simulink model "Scenario_3_PF"  (R2020b)
settings: Solver=ode1  StartTime=0.0  StopTime=10.0  RelTol=1e-3
InitFcn:
  | Scenario_3_parameters;
values from neighbouring files (symbols this model uses):
  c0 = c0_zeb    (= 6.57988e-09)    [Scenario_17_parameters_v2.m]    (also in Scenario_1_parameters_v2.m; Scenario_2_parameters_v2.m; Scenario_3_parameters_v2.m)
  c0_hawk = 6.37282e-09    [Scenario_17_parameters_v2.m]    (also in Scenario_1_parameters_v2.m; Scenario_2_parameters_v2.m; Scenario_3_parameters_v2.m)
  c1 = c1_zeb    (= 9.15905e-09)    [Scenario_17_parameters_v2.m]    (also in Scenario_1_parameters_v2.m; Scenario_2_parameters_v2.m; Scenario_3_parameters_v2.m)
  c1_hawk = 8.76156e-09    [Scenario_17_parameters_v2.m]    (also in Scenario_1_parameters_v2.m; Scenario_2_parameters_v2.m; Scenario_3_parameters_v2.m)
  fg = 50    [Scenario_17_parameters_v2.m]    (also in Scenario_1_parameters_v2.m; Scenario_2_parameters_v2.m; Scenario_3_parameters_v2.m)
  G10gen = 0.90    (= 0.9)    [Scenario_3_parameters_v2.m]
  G12gen = 0.85    [Scenario_3_parameters_v2.m]
  G1gen = 0.4692    [Scenario_17_parameters_v2.m]    (also in Scenario_1_parameters_v2.m = 0.1; Scenario_2_parameters_v2.m = 0.298581; Scenario_3_parameters_v2.m = 0.65)
  G2gen = 0.80    (= 0.8)    [Scenario_1_parameters_v2.m]    (also in Scenario_2_parameters_v2.m = 0.7; Scenario_3_parameters_v2.m = 0.4)
  G3gen = 0.85    [Scenario_1_parameters_v2.m]    (also in Scenario_2_parameters_v2.m = 0.9; Scenario_3_parameters_v2.m = 0.6)
  G4gen = 0.65    [Scenario_3_parameters_v2.m]
  G5gen = 0.75    [Scenario_17_parameters_v2.m]    (also in Scenario_1_parameters_v2.m = 0.8; Scenario_2_parameters_v2.m = 0.8; Scenario_3_parameters_v2.m = 0.705)
  G6gen = 0.90    (= 0.9)    [Scenario_17_parameters_v2.m]    (also in Scenario_1_parameters_v2.m; Scenario_2_parameters_v2.m = 0.81797; Scenario_3_parameters_v2.m = 0.45)
  G7gen = 0.20    (= 0.2)    [Scenario_17_parameters_v2.m]    (also in Scenario_1_parameters_v2.m = 0.5227; Scenario_2_parameters_v2.m = 0.5098; Scenario_3_parameters_v2.m = 0.4)
  G8gen = 0.58    [Scenario_17_parameters_v2.m]    (also in Scenario_3_parameters_v2.m = 0.65)
  G9gen = 0.8833    [Scenario_17_parameters_v2.m]    (also in Scenario_3_parameters_v2.m = 0.9)
  Ihvpk = Ihv*sqrt(2)    [Scenario_17_parameters_v2.m]    (also in Scenario_1_parameters_v2.m; Scenario_2_parameters_v2.m; Scenario_3_parameters_v2.m)
  l0 = l0_zeb    (= 0.00368)    [Scenario_17_parameters_v2.m]    (also in Scenario_1_parameters_v2.m; Scenario_2_parameters_v2.m; Scenario_3_parameters_v2.m)
  l0_hawk = 0.00373    [Scenario_17_parameters_v2.m]    (also in Scenario_1_parameters_v2.m; Scenario_2_parameters_v2.m; Scenario_3_parameters_v2.m)
  l1 = l1_zeb    (= 0.00128)    [Scenario_17_parameters_v2.m]    (also in Scenario_1_parameters_v2.m; Scenario_2_parameters_v2.m; Scenario_3_parameters_v2.m)
  L10dem = 0.04    [Scenario_3_parameters_v2.m]
  L12dem = 0.01    [Scenario_17_parameters_v2.m]    (also in Scenario_3_parameters_v2.m = 0.02)
  L13dem = 0.01    [Scenario_3_parameters_v2.m]
  l1_hawk = 0.00133    [Scenario_17_parameters_v2.m]    (also in Scenario_1_parameters_v2.m; Scenario_2_parameters_v2.m; Scenario_3_parameters_v2.m)
  L1dem = 0.25    [Scenario_17_parameters_v2.m]    (also in Scenario_3_parameters_v2.m = 0.1)
  L3dem = 0.30    (= 0.3)    [Scenario_17_parameters_v2.m]    (also in Scenario_1_parameters_v2.m = 0.1; Scenario_2_parameters_v2.m = 0.1; Scenario_3_parameters_v2.m = 0.2)
  L6dem = 0.15    [Scenario_1_parameters_v2.m]    (also in Scenario_2_parameters_v2.m; Scenario_3_parameters_v2.m = 0.1)
  L7dem = 0.10    (= 0.1)    [Scenario_1_parameters_v2.m]    (also in Scenario_2_parameters_v2.m; Scenario_3_parameters_v2.m = 0.2)
  L9dem = 0.15    [Scenario_17_parameters_v2.m]    (also in Scenario_3_parameters_v2.m = 0.1)
  Pr = Sr*PF    (= 1600500000)    [Scenario_17_parameters_v2.m]    (also in Scenario_1_parameters_v2.m = 1472500000; Scenario_2_parameters_v2.m = 1805000000; Scenario_3_parameters_v2.m = 12740000000)
  Qr = sqrt(Sr^2 - Pr^2)    [Scenario_17_parameters_v2.m]    (also in Scenario_1_parameters_v2.m; Scenario_2_parameters_v2.m; Scenario_3_parameters_v2.m)
  r0 = r0_zeb    (= 0.39362)    [Scenario_17_parameters_v2.m]    (also in Scenario_1_parameters_v2.m; Scenario_2_parameters_v2.m; Scenario_3_parameters_v2.m)
  r0_hawk = 0.44587    [Scenario_17_parameters_v2.m]    (also in Scenario_1_parameters_v2.m; Scenario_2_parameters_v2.m; Scenario_3_parameters_v2.m)
  r1 = r1_zeb    (= 0.06862)    [Scenario_17_parameters_v2.m]    (also in Scenario_1_parameters_v2.m; Scenario_2_parameters_v2.m; Scenario_3_parameters_v2.m)
  r1_hawk = 0.12087    [Scenario_17_parameters_v2.m]    (also in Scenario_1_parameters_v2.m; Scenario_2_parameters_v2.m; Scenario_3_parameters_v2.m)
  Rtpu = Xtpu/40    (= 0.0025)    [Scenario_17_parameters_v2.m]    (also in Scenario_1_parameters_v2.m = 0.00375; Scenario_2_parameters_v2.m = 0.00375; Scenario_3_parameters_v2.m)
  S10non = 500e6    (= 500000000)    [Scenario_3_parameters_v2.m]
  S12non = 250e6    (= 250000000)    [Scenario_3_parameters_v2.m]
  S1non = 700e6    (= 700000000)    [Scenario_17_parameters_v2.m]    (also in Scenario_1_parameters_v2.m = 400000000; Scenario_2_parameters_v2.m = 400000000; Scenario_3_parameters_v2.m = 1000000000)
  S2non = 300e6    (= 300000000)    [Scenario_1_parameters_v2.m]    (also in Scenario_2_parameters_v2.m; Scenario_3_parameters_v2.m = 3000000000)
  S3non = 200e6    (= 200000000)    [Scenario_1_parameters_v2.m]    (also in Scenario_2_parameters_v2.m; Scenario_3_parameters_v2.m = 1000000000)
  S4non = 2000e6    (= 2000000000)    [Scenario_3_parameters_v2.m]
  S5non = 400e6    (= 400000000)    [Scenario_17_parameters_v2.m]    (also in Scenario_1_parameters_v2.m = 500000000; Scenario_2_parameters_v2.m = 500000000; Scenario_3_parameters_v2.m = 2000000000)
  S6non = 150e6    (= 150000000)    [Scenario_17_parameters_v2.m]    (also in Scenario_1_parameters_v2.m = 400000000; Scenario_2_parameters_v2.m = 400000000; Scenario_3_parameters_v2.m = 3000000000)
  S7non = 1500e6    (= 1500000000)    [Scenario_17_parameters_v2.m]    (also in Scenario_1_parameters_v2.m = 200000000; Scenario_2_parameters_v2.m = 200000000; Scenario_3_parameters_v2.m = 4000000000)
  S8non = 600e6    (= 600000000)    [Scenario_17_parameters_v2.m]    (also in Scenario_3_parameters_v2.m = 2000000000)
  S9non = 200e6    (= 200000000)    [Scenario_17_parameters_v2.m]    (also in Scenario_3_parameters_v2.m = 1500000000)
  tonvsc = 0    [Scenario_17_parameters_v2.m]    (also in Scenario_1_parameters_v2.m; Scenario_2_parameters_v2.m; Scenario_3_parameters_v2.m = 0.0001)
  Ts = 50e-6    (= 5e-05)    [Scenario_17_parameters_v2.m]    (also in Scenario_1_parameters_v2.m = 0.0002; Scenario_2_parameters_v2.m = 2e-05; Scenario_3_parameters_v2.m = 0.0001)
  Vhv = 220e3    (= 220000)    [Scenario_17_parameters_v2.m]    (also in Scenario_1_parameters_v2.m; Scenario_2_parameters_v2.m; Scenario_3_parameters_v2.m)
  Vmv = 22e3    (= 22000)    [Scenario_17_parameters_v2.m]    (also in Scenario_1_parameters_v2.m; Scenario_2_parameters_v2.m; Scenario_3_parameters_v2.m)
  wc1 = wsw1/10    (= 848.230016469)    [Scenario_17_parameters_v2.m]    (also in Scenario_1_parameters_v2.m; Scenario_2_parameters_v2.m; Scenario_3_parameters_v2.m)
  wdc1 = wc1/10    (= 84.8230016469)    [Scenario_17_parameters_v2.m]    (also in Scenario_1_parameters_v2.m; Scenario_2_parameters_v2.m; Scenario_3_parameters_v2.m)
  wpq1 = wc1/10    (= 84.8230016469)    [Scenario_17_parameters_v2.m]    (also in Scenario_1_parameters_v2.m; Scenario_2_parameters_v2.m; Scenario_3_parameters_v2.m)
  wsw1 = ksw1*2*pi*fg    (= 8482.30016469)    [Scenario_17_parameters_v2.m]    (also in Scenario_1_parameters_v2.m; Scenario_2_parameters_v2.m; Scenario_3_parameters_v2.m)
  Xtpu = 0.10    (= 0.1)    [Scenario_17_parameters_v2.m]    (also in Scenario_1_parameters_v2.m = 0.15; Scenario_2_parameters_v2.m = 0.15; Scenario_3_parameters_v2.m)
undefined symbols (not defined in the file or in its folder): D11, Delta, Kf, r, theta0
libraries: powerlib x426, simulink_extras x305, powerlib_meascontrol x139, pid_lib x109, eeGeneralControl x72, simulink x60, eeTransforms x54, spsFirstOrderFilterLib x36, eePwmGeneratorTwoLevel x9
(part 16 of 36)

== system Scenario_3_PF/HVDC interconnection/VSC2/VSC Control/Modulation/EMT AVG ==
  note: Positive-sequence dq to abc
  note: Vref
  note: dq to abc
      | (AVG Model)
  note: negative-sequence dq to abc
  vqd+-* : Inport
  theta : Inport  Port=2
  Cartesian to Polar : simulink_extras/Transformations/Cartesian to Polar
  Cartesian to Polar1 : simulink_extras/Transformations/Cartesian to Polar
  Constant1 : Constant  Value=0
  Constant2 : Constant  Value=0
  Corrects delay : Subsystem
  Corrects delay1 : Subsystem
  Demux : Demux
  Gain : Gain  Gain=-1
  Gain2 : Gain  Gain=negseq_en
  Inverse Park Transform : eeTransforms/Inverse Park Transform  AxisAlignment=D-axis  PowerInvariant=off
  Inverse Park Transform1 : eeTransforms/Inverse Park Transform  AxisAlignment=D-axis  PowerInvariant=off
  Mux1 : Mux  Inputs=3
  Mux2 : Mux  Inputs=3
  Polar to Cartesian : simulink_extras/Transformations/Polar to Cartesian
      settings: SourceProductBaseCode=SL
  Polar to Cartesian1 : simulink_extras/Transformations/Polar to Cartesian
      settings: SourceProductBaseCode=SL
  Sum : Sum
  Sum1 : Sum  Inputs=|++
  Sum4 : Sum  Inputs=|++
  Unit Delay : UnitDelay  SampleTime=-1  HasFrameUpgradeWarning=on
  Ref : Outport
  wires:
  Demux/3 -> [vqnref]
  Demux/1 -> [vqpref]
  Demux/4 -> [vdnref]
  Demux/2 -> [vdpref]
  vqd+-*/1 -> Demux/1
  Gain2/1 -> Sum/2
  Polar to Cartesian/2 -> Mux1/2
  Sum4/1 -> Polar to Cartesian/2
  Mux1/1 -> Inverse Park Transform/1
  Cartesian to Polar/1 -> Polar to Cartesian/1
  [vdpref] -> Cartesian to Polar/1
  Cartesian to Polar/2 -> Sum4/1
  Constant1/1 -> Mux1/3
  [vqpref] -> Cartesian to Polar/2
  Corrects delay/1(dphi) -> Sum4/2
  Polar to Cartesian/1 -> Mux1/1
  Unit Delay/1 -> Ref/1
  [vdnref] -> Cartesian to Polar1/1
  Mux2/1 -> Inverse Park Transform1/1
  Cartesian to Polar1/1 -> Polar to Cartesian1/1
  Constant2/1 -> Mux2/3
  Polar to Cartesian1/2 -> Mux2/2
  Sum1/1 -> Polar to Cartesian1/2
  [vqnref] -> Cartesian to Polar1/2
  Corrects delay1/1(dphi) -> Sum1/2
  Gain/1 -> Inverse Park Transform1/2
  Polar to Cartesian1/1 -> Mux2/1
  Cartesian to Polar1/2 -> Sum1/1
  theta/1 -> Gain/1, Inverse Park Transform/2
  Sum/1 -> Unit Delay/1
  Inverse Park Transform/1 -> Sum/1
  Inverse Park Transform1/1 -> Gain2/1

== system Scenario_3_PF/HVDC interconnection/VSC2/VSC Control/Modulation/EMT Switching ==
  note: Interpolate pulses
  note: Pulses
  note: Modulation
  note: negative-sequence dq to abc
  note: Positive-sequence dq to abc
  vqd+-* : Inport
  theta : Inport  Port=2
  Cartesian to Polar : simulink_extras/Transformations/Cartesian to Polar
  Cartesian to Polar1 : simulink_extras/Transformations/Cartesian to Polar
  Constant : Constant  Value=0
  Constant1 : Constant  Commented=on  Value=Vdc
  Constant2 : Constant  Value=0
  Corrects delay : Subsystem
  Corrects delay1 : Subsystem
  Demux : Demux
  Gain : Gain  Gain=1/(Vdc/2)
  Gain1 : Gain  Gain=-1
  Gain2 : Gain  Gain=negseq_en
  Inverse Park Transform1 : eeTransforms/Inverse Park Transform  AxisAlignment=D-axis  PowerInvariant=off
  Inverse Park Transform2 : eeTransforms/Inverse Park Transform  AxisAlignment=D-axis  PowerInvariant=off
  Mux : Mux  Inputs=3
  Mux1 : Mux  Inputs=3
  Mux2 : Mux  Inputs=3
  PWM Generator (Interpolation)1 : powerlib_meascontrol/Pulse & Signal Generators/PWM Generator (Interpolation)  GeneratorType=Two-level, three-phase  Fc=ksw*fg  InitialPhase=0  Ts=Ts
      settings: SourceProductBaseCode=PS
  "PWM Generator (Three-phase, Two-level)" : eePwmGeneratorTwoLevel/PWM Generator (Three-phase, Two-level)  Commented=on  PWMMode=Continuous PWM (CPWM)  CPWMMode=SPWM: sinusoidal PWM  DPWMMode=60 DPWM: 60 degree discontinuous PWM  fsw=ksw*fg  Ts=Ts
      settings: SourceProductBaseCode=PS
  Polar to Cartesian : simulink_extras/Transformations/Polar to Cartesian
      settings: SourceProductBaseCode=SL
  Polar to Cartesian1 : simulink_extras/Transformations/Polar to Cartesian
      settings: SourceProductBaseCode=SL
  Sum : Sum
  Sum1 : Sum  Inputs=|++
  Sum4 : Sum  Inputs=|++
  Unit Delay : UnitDelay  SampleTime=-1  HasFrameUpgradeWarning=on
  Ref : Outport
  wires:
  [vqpref] -> Cartesian to Polar/2
  Demux/4 -> [vdnref]
  Demux/3 -> [vqnref]
  Demux/2 -> [vdpref]
  Demux/1 -> [vqpref]
  vqd+-*/1 -> Demux/1
  Mux1/1 -> Unit Delay/1
  Sum/1 -> Gain/1
  Unit Delay/1 -> Ref/1
  PWM Generator (Interpolation)1/2 -> Mux1/2
  PWM Generator (Interpolation)1/1 -> Mux1/1
  PWM Generator (Interpolation)1/3 -> Mux1/3
  Gain/1 -> PWM Generator (Interpolation)1/1
  Constant1/1 -> "PWM Generator (Three-phase, Two-level)"/2
  theta/1 -> Inverse Park Transform2/2, Gain1/1
  Gain2/1 -> Sum/2
  Constant/1 -> Mux/3
  Cartesian to Polar/2 -> Sum4/1
  Sum4/1 -> Polar to Cartesian/2
  Corrects delay/1(dphi) -> Sum4/2
  Cartesian to Polar/1 -> Polar to Cartesian/1
  Mux/1 -> Inverse Park Transform2/1
  Polar to Cartesian/1 -> Mux/1
  Polar to Cartesian/2 -> Mux/2
  [vdpref] -> Cartesian to Polar/1
  Mux2/1 -> Inverse Park Transform1/1
  Sum1/1 -> Polar to Cartesian1/2
  Inverse Park Transform2/1 -> Sum/1
  Corrects delay1/1(dphi) -> Sum1/2
  Polar to Cartesian1/2 -> Mux2/2
  Cartesian to Polar1/1 -> Polar to Cartesian1/1
  Cartesian to Polar1/2 -> Sum1/1
  Polar to Cartesian1/1 -> Mux2/1
  [vdnref] -> Cartesian to Polar1/1
  [vqnref] -> Cartesian to Polar1/2
  Inverse Park Transform1/1 -> Gain2/1
  Constant2/1 -> Mux2/3
  Gain1/1 -> Inverse Park Transform1/2

== system Scenario_3_PF/HVDC interconnection/VSC2/VSC Control/Modulation/Phasor I and Phasor PQ ==
  note: Negative-sequence dq to abc
  note: Positive-sequence dq to abc
  note: dq to abc
      | (Phasor I and Phasor PQ)
  iqd+-* : Inport
  theta : Inport  Port=2
  Constant : Constant  Commented=on  Value=negseq_en
  Constant1 : Constant  Value=complex(0,0)
  Delay : Delay  DelayLength=1
  Demux3 : Demux
  Display : Display  Commented=on
  Exp : Math  OutputSignalType=complex  SaturateOnIntegerOverflow=on
  Exp1 : Math  OutputSignalType=complex  SaturateOnIntegerOverflow=on
  Gain : Gain  Gain=-1
  Gain1 : Gain  Gain=1i
  Gain2 : Gain  Gain=exp(1i*pi/6)
  Gain3 : Gain  Gain=exp(-1i*pi/6)
  Gain5 : Gain  Gain=1i
  Gain7 : Gain  Gain=negseq_en
  Gain8 : Gain  Gain=-1
  Gain9 : Gain  Gain=-1
  Inverse Park Transform (Phasor) : Subsystem  Commented=on
  Mux3 : Mux  Inputs=3
  Product : Product
  Product1 : Product
  RL time constant : Subsystem  Commented=through  mask{R=Rt, L=Lt, f=fg}
      mask prompts: R "Series resistance (R)"; L "Series inductance (L)"; f "Power frequency (Hz)"
      mask init:
      | w = 2*pi*f;
  Real-Imag to Complex : RealImagToComplex
  Real-Imag to Complex1 : RealImagToComplex
  Subsystem : Subsystem
      mask init:
      | a = exp(1i*2*pi/3);
      | a2 = exp(1i*4*pi/3);
  Ref : Outport
  wires:
  Demux3/4 -> [idnref]
  iqd+-*/1 -> Demux3/1
  Demux3/1 -> [iqpref]
  Demux3/2 -> [idpref]
  Demux3/3 -> [iqnref]
  Constant/1 -> Display/1
  Gain/1 -> Real-Imag to Complex/2
  [idpref] -> Gain/1
  Exp1/1 -> Product1/1
  Real-Imag to Complex1/1 -> Product1/2
  Gain1/1 -> Exp1/1
  Constant1/1 -> Mux3/1
  Mux3/1 -> Subsystem/1(012)
  Product/1 -> Gain2/1
  Real-Imag to Complex/1 -> Product/1
  [iqpref] -> Real-Imag to Complex/1
  Exp/1 -> Product/2
  Gain5/1 -> Exp/1
  theta/1 -> Gain1/1, Gain5/1
  Delay/1 -> Ref/1
  Subsystem/1(abc) -> Delay/1
  Gain3/1 -> Mux3/3
  Product1/1 -> Gain7/1
  Gain7/1 -> Gain3/1
  [idnref] -> Gain8/1
  [iqnref] -> Gain9/1
  Gain9/1 -> Real-Imag to Complex1/1
  Gain8/1 -> Real-Imag to Complex1/2
  Gain2/1 -> Mux3/2

== system Scenario_3_PF/HVDC interconnection/VSC2/VSC Control/Modulation/Phasor Quasi-EMT ==
  note: dq to abc
      | (Phasor)
  note: Positive-sequence dq to abc
  note: Negative-sequence dq to abc
  vqd+-* : Inport
  theta : Inport  Port=2
  vqd+- : Inport  Port=3
  Cartesian to Polar : simulink_extras/Transformations/Cartesian to Polar
  Cartesian to Polar1 : simulink_extras/Transformations/Cartesian to Polar
  Constant : Constant  Commented=on  Value=negseq_en
  Constant1 : Constant  Value=complex(0,0)
  Corrects delay : Subsystem  Commented=on
  Corrects delay2 : Subsystem  Commented=on
  Delay : Delay  DelayLength=1
  Demux : Demux  Outputs=2
  Demux1 : Demux  Outputs=2
  Demux2 : Demux
  Demux3 : Demux
  Display : Display  Commented=on
  Exp : Math  OutputSignalType=complex  SaturateOnIntegerOverflow=on
  Exp1 : Math  OutputSignalType=complex  SaturateOnIntegerOverflow=on
  Gain : Gain  Gain=-1
  Gain1 : Gain  Gain=1i
  Gain2 : Gain  Gain=exp(1i*pi/6)
  Gain3 : Gain  Gain=exp(-1i*pi/6)
  Gain5 : Gain  Gain=1i
  Gain7 : Gain  Gain=negseq_en
  Gain8 : Gain  Gain=-1
  Gain9 : Gain  Gain=-1
  Inverse Park Transform (Phasor) : Subsystem  Commented=on
  Mux{,1..2,4} (4 alike) : Mux  Inputs=2
  Mux3 : Mux  Inputs=3
  Polar to Cartesian : simulink_extras/Transformations/Polar to Cartesian
      settings: SourceProductBaseCode=SL
  Polar to Cartesian1 : simulink_extras/Transformations/Polar to Cartesian
      settings: SourceProductBaseCode=SL
  Product : Product
  Product1 : Product
  Real-Imag to Complex : RealImagToComplex
  Real-Imag to Complex1 : RealImagToComplex
  Subsystem : Subsystem
      mask init:
      | a = exp(1i*2*pi/3);
      | a2 = exp(1i*4*pi/3);
  Sum1 : Sum  Inputs=|++
  Sum4 : Sum  Inputs=|++
  V to I RL (+seq) : Subsystem  mask{R=Rt, L=Lt, f=fg}
      mask prompts: R "Series resistance (R)"; L "Series inductance (L)"; f "Power frequency (Hz)"
      mask init:
      | w = 2*pi*f;
  V to I RL (- seq) : Subsystem  mask{R=Rt, L=Lt, f=fg}
      mask prompts: R "Series resistance (R)"; L "Series inductance (L)"; f "Power frequency (Hz)"
      mask init:
      | w = 2*pi*f;
  Ref : Outport
  wires:
  Demux3/3 -> [vqnref]
  Demux3/4 -> [vdnref]
  Demux3/1 -> [vqpref]
  vqd+-*/1 -> Demux3/1
  Demux3/2 -> [vdpref]
  Gain2/1 -> Mux3/2
  Gain8/1 -> Real-Imag to Complex1/2
  Gain9/1 -> Real-Imag to Complex1/1
  Demux1/2 -> Gain9/1
  Demux1/1 -> Gain8/1
  Gain7/1 -> Gain3/1
  Product1/1 -> Gain7/1
  Gain3/1 -> Mux3/3
  Subsystem/1(abc) -> Delay/1
  Delay/1 -> Ref/1
  Cartesian to Polar1/1 -> Polar to Cartesian1/1
  theta/1 -> Gain5/1, Gain1/1
  [vqp] -> Mux1/2
  V to I RL (+seq)/1(idIq) -> Demux/1
  Gain5/1 -> Exp/1
  Exp/1 -> Product/2
  Demux/2 -> Real-Imag to Complex/1
  Real-Imag to Complex/1 -> Product/1
  Product/1 -> Gain2/1
  Mux3/1 -> Subsystem/1(012)
  Constant1/1 -> Mux3/1
  Sum4/1 -> Polar to Cartesian/2
  Cartesian to Polar/1 -> Polar to Cartesian/1
  Cartesian to Polar/2 -> Sum4/1
  Corrects delay/1(dphi) -> Sum4/2
  Polar to Cartesian/1 -> Mux/1
  Polar to Cartesian/2 -> Mux/2
  [vdpref] -> Cartesian to Polar/1
  [vqpref] -> Cartesian to Polar/2
  Mux/1 -> V to I RL (+seq)/2(Vdq2)
  Mux1/1 -> V to I RL (+seq)/1(Vdq1)
  [vdnref] -> Cartesian to Polar1/1
  Sum1/1 -> Polar to Cartesian1/2
  [vqnref] -> Cartesian to Polar1/2
  Polar to Cartesian1/2 -> Mux2/2
  Polar to Cartesian1/1 -> Mux2/1
  Cartesian to Polar1/2 -> Sum1/1
  Corrects delay2/1(dphi) -> Sum1/2
  Mux2/1 -> V to I RL (- seq)/2(Vdq2)
  Mux4/1 -> V to I RL (- seq)/1(Vdq1)
  [vqn] -> Mux4/2
  [vdn] -> Mux4/1
  V to I RL (- seq)/1(idIq) -> Demux1/1
  Gain1/1 -> Exp1/1
  Real-Imag to Complex1/1 -> Product1/2
  Exp1/1 -> Product1/1
  vqd+-/1 -> Demux2/1
  Demux2/2 -> [vdp]
  Demux2/3 -> [vqn]
  Demux2/4 -> [vdn]
  Demux2/1 -> [vqp]
  [vdp] -> Mux1/1
  Demux/1 -> Gain/1
  Gain/1 -> Real-Imag to Complex/2
  Constant/1 -> Display/1

== system Scenario_3_PF/G1/VSC/VSC Control/Control loops/Phasor I 1st/Inner-loop ==
  note: Positive-sequence current
  note: Negative-sequence current
  iq+* : Inport
  id+* : Inport  Port=2
  iq-* : Inport  Port=3
  id-* : Inport  Port=4
  First-Order Filter{,1..3} (4 alike) : powerlib_meascontrol/Filters/First-Order Filter  FilterType=Lowpass  Tc=1/wc  Ts=0  Initialize=off  Vac_Init=[0, 0, 60]  Vdc_Init=0  PlotResponse=off  FreqRange="[0,  200,  1]"
  iq+ref : Outport
  id+ref : Outport  Port=2
  iq-ref : Outport  Port=3
  id-ref : Outport  Port=4
  wires:
  First-Order Filter3/1 -> id-ref/1
  id-*/1 -> First-Order Filter3/1
  First-Order Filter2/1 -> iq-ref/1
  iq-*/1 -> First-Order Filter2/1
  First-Order Filter1/1 -> id+ref/1
  id+*/1 -> First-Order Filter1/1
  First-Order Filter/1 -> iq+ref/1
  iq+*/1 -> First-Order Filter/1

== system Scenario_3_PF/G1/VSC/VSC Control/Control loops/Phasor I 1st/Outer-loop ==
  note: Limits the converter current
  note: Frequency droop
  note: Voltage droop
  note: Reactive power control
  note: Active power control
  note: LVRT
  Pset : Inport
  Qset : Inport  Port=2
  vqd+- : Inport  Port=3
  iqd+- : Inport  Port=4
  freq : Inport  Port=5
  Blk : Inport  Port=6
  Cartesian to Polar : simulink_extras/Transformations/Cartesian to Polar
  Compare To Constant1 : simulink/Logic and Bit Operations/Compare To Constant  relop=<  const=0  OutDataTypeStr=boolean
  Constant1 : Constant  Value=fg
  Constant10 : Constant  Value=0
  Constant11 : Constant  Value=Vlvrt0
  Constant2 : Constant  Value=Vmvpk
  Constant9 : Constant  Value=0
  Demux : Demux  Outputs=2
  Demux1 : Demux
  Demux2 : Demux
  Gain14 : Gain  Gain=1/Vmvpk
  Gain15 : Gain  Gain=Klvrt
  Gain16 : Gain  Gain=Iconvbase
  Gain5 : Gain  Gain=-1/Kfdroop*(Pconv/fg)
  Gain6 : Gain  Gain=-1/Kvdroop*(Pconv/Vmvpk)
  Mux1 : Mux  Inputs=10
  NOT : Logic  Operator=NOT  IconShape=distinctive  AllPortsSameDT=off  OutDataTypeStr=boolean
  PID Controller1 : pid_lib/PID Controller  Controller=PI  Form=Ideal  TimeDomain=Continuous-time  UseExternalTs=off  SampleTime=-1  IntegratorMethod=Forward Euler  FilterMethod=Forward Euler  ControllerParametersSource=internal  P=kp_pq  I=1/ti_pq  D=0  UseFilter=on  N=100  TunerSelectOption=Transfer Function Based (PID Tuner App)  InitialConditionSource=internal  InitialConditionForIntegrator=0  InitialConditionForFilter=0  DifferentiatorICPrevScaledInput=0  ExternalReset=none  TrackingMode=off  Kt=1  LimitOutput=off  SatLimitsSource=internal  UpperSaturationLimit=inf  LowerSaturationLimit=-inf  LinearizeAsGain=on  AntiWindupMode=none  Kb=1  POutMin=[]  POutMax=[]  IOutMin=[]  IOutMax=[]  DOutMin=[]  DOutMax=[]  NOutMin=[]  NOutMax=[]  SumOutMin=[]  SumOutMax=[]  SaturationOutMin=[]  SaturationOutMax=[]  PParamMin=[]  PParamMax=[]  IParamMin=[]  IParamMax=[]  DParamMin=[]  DParamMax=[]  NParamMin=[]  NParamMax=[]  KbParamMin=[]  KbParamMax=[]  KtParamMin=[]  KtParamMax=[]  KbOutMin=[]  KbOutMax=[]  KtOutMin=[]  KtOutMax=[]  IntegratorOutMin=[]  IntegratorOutMax=[]  FilterOutMin=[]  FilterOutMax=[]  SumI1OutMin=[]  SumI1OutMax=[]  SumI2OutMin=[]  SumI2OutMax=[]  SumI3OutMin=[]  SumI3OutMax=[]  SumI4OutMin=[]  SumI4OutMax=[]  SumDOutMin=[]  SumDOutMax=[]  DifferentiatorOutMin=[]  DifferentiatorOutMax=[]  FilterDiffOutCoefMin=[]  FilterDiffOutCoefMax=[]  ReciprocalOutMin=[]  ReciprocalOutMax=[]  SumDenOutMin=[]  SumDenOutMax=[]  SumNumOutMin=[]  SumNumOutMax=[]  DivideOutMin=[]  DivideOutMax=[]  UdiffTsProdOutMin=[]  UdiffTsProdOutMax=[]  NTsProdOutMin=[]  NTsProdOutMax=[]  UintegralTsProdOutMin=[]  UintegralTsProdOutMax=[]  UngainTsProdOutMin=[]  UngainTsProdOutMax=[]  IntegratorContinuousStateAttributes=''  IntegratorStateMustResolveToSignalObject=off  IntegratorRTWStateStorageClass=Auto  FilterContinuousStateAttributes=''  FilterStateMustResolveToSignalObject=off  FilterRTWStateStorageClass=Auto  ParallelPVariant=Passthrough  IdealPVariant=InternalParameters  IVariant=InternalParameters  DVariant=Disabled  IntegratorVariant=Continuous  SatVariant=Disabled  AWVariant=Passthrough  PCopyVariant=Disabled  TRVariant=Disabled  FdbkBlocksVariant=Forward  IdealPFdbkVariant=Disabled  SatFdbkVariant=Disabled  DerivativeFilterVariant=Disabled  NVariant=Disabled  NCopyVariant=Disabled_SignalSpec  FilterICVariant=Disabled  IntegratorICVariant=InternalICs  ExternalResetVariant=Disabled  TRSumVariant=Passthrough  SumFdbkVariant=Disabled  SumVariant=Sum_PI  TsampFilterVariant=InternalTs  TsampNgainVariant=Passthrough  TsampIntegralVariant=Passthrough  ExternalSaturationOutDataTypeStr=Inherit: Same as second input
  PID Controller6 : pid_lib/PID Controller  Controller=PI  Form=Ideal  TimeDomain=Continuous-time  UseExternalTs=off  SampleTime=-1  IntegratorMethod=Forward Euler  FilterMethod=Forward Euler  ControllerParametersSource=internal  P=kp_pq  I=1/ti_pq  D=0  UseFilter=on  N=100  TunerSelectOption=Transfer Function Based (PID Tuner App)  InitialConditionSource=internal  InitialConditionForIntegrator=0  InitialConditionForFilter=0  DifferentiatorICPrevScaledInput=0  ExternalReset=none  TrackingMode=off  Kt=1  LimitOutput=off  SatLimitsSource=internal  UpperSaturationLimit=inf  LowerSaturationLimit=-inf  LinearizeAsGain=on  AntiWindupMode=none  Kb=1  POutMin=[]  POutMax=[]  IOutMin=[]  IOutMax=[]  DOutMin=[]  DOutMax=[]  NOutMin=[]  NOutMax=[]  SumOutMin=[]  SumOutMax=[]  SaturationOutMin=[]  SaturationOutMax=[]  PParamMin=[]  PParamMax=[]  IParamMin=[]  IParamMax=[]  DParamMin=[]  DParamMax=[]  NParamMin=[]  NParamMax=[]  KbParamMin=[]  KbParamMax=[]  KtParamMin=[]  KtParamMax=[]  KbOutMin=[]  KbOutMax=[]  KtOutMin=[]  KtOutMax=[]  IntegratorOutMin=[]  IntegratorOutMax=[]  FilterOutMin=[]  FilterOutMax=[]  SumI1OutMin=[]  SumI1OutMax=[]  SumI2OutMin=[]  SumI2OutMax=[]  SumI3OutMin=[]  SumI3OutMax=[]  SumI4OutMin=[]  SumI4OutMax=[]  SumDOutMin=[]  SumDOutMax=[]  DifferentiatorOutMin=[]  DifferentiatorOutMax=[]  FilterDiffOutCoefMin=[]  FilterDiffOutCoefMax=[]  ReciprocalOutMin=[]  ReciprocalOutMax=[]  SumDenOutMin=[]  SumDenOutMax=[]  SumNumOutMin=[]  SumNumOutMax=[]  DivideOutMin=[]  DivideOutMax=[]  UdiffTsProdOutMin=[]  UdiffTsProdOutMax=[]  NTsProdOutMin=[]  NTsProdOutMax=[]  UintegralTsProdOutMin=[]  UintegralTsProdOutMax=[]  UngainTsProdOutMin=[]  UngainTsProdOutMax=[]  IntegratorContinuousStateAttributes=''  IntegratorStateMustResolveToSignalObject=off  IntegratorRTWStateStorageClass=Auto  FilterContinuousStateAttributes=''  FilterStateMustResolveToSignalObject=off  FilterRTWStateStorageClass=Auto  ParallelPVariant=Passthrough  IdealPVariant=InternalParameters  IVariant=InternalParameters  DVariant=Disabled  IntegratorVariant=Continuous  SatVariant=Disabled  AWVariant=Passthrough  PCopyVariant=Disabled  TRVariant=Disabled  FdbkBlocksVariant=Forward  IdealPFdbkVariant=Disabled  SatFdbkVariant=Disabled  DerivativeFilterVariant=Disabled  NVariant=Disabled  NCopyVariant=Disabled_SignalSpec  FilterICVariant=Disabled  IntegratorICVariant=InternalICs  ExternalResetVariant=Disabled  TRSumVariant=Passthrough  SumFdbkVariant=Disabled  SumVariant=Sum_PI  TsampFilterVariant=InternalTs  TsampNgainVariant=Passthrough  TsampIntegralVariant=Passthrough  ExternalSaturationOutDataTypeStr=Inherit: Same as second input
  Polar to Cartesian : simulink_extras/Transformations/Polar to Cartesian
      settings: SourceProductBaseCode=SL
  Power calculation : Subsystem
  Product3 : Product
  Saturation : Saturate  UpperLimit=Imax  LowerLimit=0
  Saturation1 : Saturate  UpperLimit=0.1*Pconv  LowerLimit=-0.1*Pconv
  Saturation2 : Saturate  UpperLimit=0.1*Pconv  LowerLimit=-0.1*Pconv
  Saturation7 : Saturate  UpperLimit=0  LowerLimit=-Qmax_lvrt
  Second-Order Filter : eeGeneralControl/Second-Order Filter  FilterType=Low-pass  fn=150  Zeta=0.9  Ts=-1  A0=0  Ph0=0  f0=0  b0=0
      settings: SourceProductBaseCode=PS
  Second-Order Filter1 : eeGeneralControl/Second-Order Filter  FilterType=Low-pass  fn=10  Zeta=0.9  Ts=-1  A0=50  Ph0=0  f0=0.001  b0=50
      settings: SourceProductBaseCode=PS
  Step : Step  Commented=on  Time=0.1  After=0.3*3711  SampleTime=0
  Step1 : Step  Commented=on  Time=0.2  After=0.2*3711  SampleTime=0
  Sum{,4,6,11} (4 alike) : Sum  Inputs=|+-
  Sum2 : Sum  Inputs=-+|
  Sum3 : Sum  Inputs=|++
  Sum5 : Sum  Inputs=|++
  Switch2 : Switch  Threshold=1
  Terminator : Terminator
  iq+* : Outport
  id+* : Outport  Port=2
  iq-* : Outport  Port=3
  id-* : Outport  Port=4
  m : Outport  Port=5
  wires:
  Constant10/1 -> id-*/1
  Constant9/1 -> iq-*/1
  Second-Order Filter1/1 -> Sum4/2
  [f] -> Second-Order Filter1/1
  Saturation2/1 -> Sum5/2
  Qset/1 -> Sum5/1
  Cartesian to Polar/2 -> Polar to Cartesian/2
  Polar to Cartesian/1 -> iq+*/1
  Polar to Cartesian/2 -> id+*/1
  Cartesian to Polar/1 -> Saturation/1
  Saturation/1 -> Polar to Cartesian/1
  Demux/1 -> Sum/2  "P"
  Demux/2 -> Sum2/1  "Q"
  Sum3/1 -> Sum/1  "Pref"
  Constant1/1 -> Sum4/1
  Gain5/1 -> Saturation1/1
  Sum4/1 -> Gain5/1
  Saturation1/1 -> Sum3/2
  Sum5/1 -> Sum2/2  "Qref"
  Sum6/1 -> Gain6/1
  Gain6/1 -> Saturation2/1
  [vqfilt] -> Sum6/2
  Constant2/1 -> Sum6/1
  Sum2/1 -> Product3/1
  Pset/1 -> Sum3/1
  PID Controller1/1 -> Cartesian to Polar/1
  Blk/1 -> Terminator/1
  freq/1 -> [f]
  [vqp] -> Mux1/1
  Mux1/1 -> m/1
  Product3/1 -> PID Controller6/1
  Sum/1 -> PID Controller1/1
  Second-Order Filter/1 -> [vqfilt]
  vqd+-/1 -> Demux1/1
  iqd+-/1 -> Demux2/1
  Demux1/1 -> Second-Order Filter/1, [vqp]
  Demux1/2 -> [vdp]
  Demux1/3 -> [vqn]
  Demux1/4 -> [vdn]
  Demux2/1 -> [iqp]
  Demux2/2 -> [idp]
  Demux2/3 -> [iqn]
  Demux2/4 -> [idn]
  [vqp] -> Power calculation/1(vq+)
  [iqp] -> Power calculation/3(iq+)
  Power calculation/1(PQ) -> [PQdq], Demux/1
  [idp] -> Power calculation/4(id+)
  [vdp] -> Power calculation/2(vd+)
  [vqn] -> Power calculation/5(vq-)
  [vdn] -> Power calculation/6(vd-)
  [iqn] -> Power calculation/7(iq-)
  [idn] -> Power calculation/8(id-)
  [LVRT_true] -> NOT/1
  NOT/1 -> Product3/2
  [LVRT_true] -> Switch2/2
  PID Controller6/1 -> Switch2/3
  Switch2/1 -> Cartesian to Polar/2
  Compare To Constant1/1 -> [LVRT_true]
  Gain16/1 -> Switch2/1
  Gain15/1 -> Saturation7/1
  Saturation7/1 -> Compare To Constant1/1, Gain16/1
  [vqfilt] -> Gain14/1
  Sum11/1 -> Gain15/1
  Gain14/1 -> Sum11/2
  Constant11/1 -> Sum11/1
  [vdp] -> Mux1/2
  [vqn] -> Mux1/3
  [vdn] -> Mux1/4
  [iqn] -> Mux1/7
  [idn] -> Mux1/8
  [f] -> Mux1/9
  [PQdq] -> Mux1/10
  [idp] -> Mux1/6
  [iqp] -> Mux1/5

== system Scenario_3_PF/G1/VSC/VSC Control/Control loops/Phasor I ref/Outer-loop ==
  note: LVRT
  note: Active power control
  note: Reactive power control
  note: Voltage droop
  note: Frequency droop
  note: Limits the converter current
  Pset : Inport
  Qset : Inport  Port=2
  vqd+- : Inport  Port=3
  iqd+- : Inport  Port=4
  freq : Inport  Port=5
  Blk : Inport  Port=6
  Cartesian to Polar : simulink_extras/Transformations/Cartesian to Polar
  Compare To Constant1 : simulink/Logic and Bit Operations/Compare To Constant  relop=<  const=0  OutDataTypeStr=boolean
  Constant1 : Constant  Value=fg
  Constant10 : Constant  Value=0
  Constant11 : Constant  Value=Vlvrt0
  Constant2 : Constant  Value=Vmvpk
  Constant9 : Constant  Value=0
  Demux : Demux  Outputs=2
  Demux1 : Demux
  Demux2 : Demux
  Gain : Gain  Gain=2/3 * 1/Vmvpk * wpq
  Gain1 : Gain  Gain=2/3 * 1/Vmvpk * wpq
  Gain14 : Gain  Gain=1/Vmvpk
  Gain15 : Gain  Gain=Klvrt
  Gain16 : Gain  Gain=Iconvbase
  Gain5 : Gain  Gain=-1/Kfdroop*(Pconv/fg)
  Gain6 : Gain  Gain=-1/Kvdroop*(Pconv/Vmvpk)
  Integrator : Integrator
  Integrator1 : Integrator
  Mux1 : Mux  Inputs=10
  NOT : Logic  Operator=NOT  IconShape=distinctive  AllPortsSameDT=off  OutDataTypeStr=boolean
  PID Controller1 : pid_lib/PID Controller  Commented=on  Controller=I  Form=Ideal  TimeDomain=Continuous-time  UseExternalTs=off  SampleTime=-1  IntegratorMethod=Forward Euler  FilterMethod=Forward Euler  ControllerParametersSource=internal  P=kp_pq  I=1/wpq  D=0  UseFilter=on  N=100  TunerSelectOption=Transfer Function Based (PID Tuner App)  InitialConditionSource=internal  InitialConditionForIntegrator=0  InitialConditionForFilter=0  DifferentiatorICPrevScaledInput=0  ExternalReset=none  TrackingMode=off  Kt=1  LimitOutput=off  SatLimitsSource=internal  UpperSaturationLimit=inf  LowerSaturationLimit=-inf  LinearizeAsGain=on  AntiWindupMode=none  Kb=1  POutMin=[]  POutMax=[]  IOutMin=[]  IOutMax=[]  DOutMin=[]  DOutMax=[]  NOutMin=[]  NOutMax=[]  SumOutMin=[]  SumOutMax=[]  SaturationOutMin=[]  SaturationOutMax=[]  PParamMin=[]  PParamMax=[]  IParamMin=[]  IParamMax=[]  DParamMin=[]  DParamMax=[]  NParamMin=[]  NParamMax=[]  KbParamMin=[]  KbParamMax=[]  KtParamMin=[]  KtParamMax=[]  KbOutMin=[]  KbOutMax=[]  KtOutMin=[]  KtOutMax=[]  IntegratorOutMin=[]  IntegratorOutMax=[]  FilterOutMin=[]  FilterOutMax=[]  SumI1OutMin=[]  SumI1OutMax=[]  SumI2OutMin=[]  SumI2OutMax=[]  SumI3OutMin=[]  SumI3OutMax=[]  SumI4OutMin=[]  SumI4OutMax=[]  SumDOutMin=[]  SumDOutMax=[]  DifferentiatorOutMin=[]  DifferentiatorOutMax=[]  FilterDiffOutCoefMin=[]  FilterDiffOutCoefMax=[]  ReciprocalOutMin=[]  ReciprocalOutMax=[]  SumDenOutMin=[]  SumDenOutMax=[]  SumNumOutMin=[]  SumNumOutMax=[]  DivideOutMin=[]  DivideOutMax=[]  UdiffTsProdOutMin=[]  UdiffTsProdOutMax=[]  NTsProdOutMin=[]  NTsProdOutMax=[]  UintegralTsProdOutMin=[]  UintegralTsProdOutMax=[]  UngainTsProdOutMin=[]  UngainTsProdOutMax=[]  IntegratorContinuousStateAttributes=''  IntegratorStateMustResolveToSignalObject=off  IntegratorRTWStateStorageClass=Auto  FilterContinuousStateAttributes=''  FilterStateMustResolveToSignalObject=off  FilterRTWStateStorageClass=Auto  ParallelPVariant=Disabled  IdealPVariant=Disabled  IVariant=InternalParameters  DVariant=Disabled  IntegratorVariant=Continuous  SatVariant=Disabled  AWVariant=Passthrough  PCopyVariant=Disabled  TRVariant=Disabled  FdbkBlocksVariant=Forward  IdealPFdbkVariant=Disabled  SatFdbkVariant=Disabled  DerivativeFilterVariant=Disabled  NVariant=Disabled  NCopyVariant=Disabled_SignalSpec  FilterICVariant=Disabled  IntegratorICVariant=InternalICs  ExternalResetVariant=Disabled  TRSumVariant=Passthrough  SumFdbkVariant=Disabled  SumVariant=Passthrough_I  TsampFilterVariant=InternalTs  TsampNgainVariant=Passthrough  TsampIntegralVariant=Passthrough  ExternalSaturationOutDataTypeStr=Inherit: Same as second input
  PID Controller6 : pid_lib/PID Controller  Commented=on  Controller=I  Form=Ideal  TimeDomain=Continuous-time  UseExternalTs=off  SampleTime=-1  IntegratorMethod=Forward Euler  FilterMethod=Forward Euler  ControllerParametersSource=internal  P=kp_pq  I=1/wpq  D=0  UseFilter=on  N=100  TunerSelectOption=Transfer Function Based (PID Tuner App)  InitialConditionSource=internal  InitialConditionForIntegrator=0  InitialConditionForFilter=0  DifferentiatorICPrevScaledInput=0  ExternalReset=none  TrackingMode=off  Kt=1  LimitOutput=off  SatLimitsSource=internal  UpperSaturationLimit=inf  LowerSaturationLimit=-inf  LinearizeAsGain=on  AntiWindupMode=none  Kb=1  POutMin=[]  POutMax=[]  IOutMin=[]  IOutMax=[]  DOutMin=[]  DOutMax=[]  NOutMin=[]  NOutMax=[]  SumOutMin=[]  SumOutMax=[]  SaturationOutMin=[]  SaturationOutMax=[]  PParamMin=[]  PParamMax=[]  IParamMin=[]  IParamMax=[]  DParamMin=[]  DParamMax=[]  NParamMin=[]  NParamMax=[]  KbParamMin=[]  KbParamMax=[]  KtParamMin=[]  KtParamMax=[]  KbOutMin=[]  KbOutMax=[]  KtOutMin=[]  KtOutMax=[]  IntegratorOutMin=[]  IntegratorOutMax=[]  FilterOutMin=[]  FilterOutMax=[]  SumI1OutMin=[]  SumI1OutMax=[]  SumI2OutMin=[]  SumI2OutMax=[]  SumI3OutMin=[]  SumI3OutMax=[]  SumI4OutMin=[]  SumI4OutMax=[]  SumDOutMin=[]  SumDOutMax=[]  DifferentiatorOutMin=[]  DifferentiatorOutMax=[]  FilterDiffOutCoefMin=[]  FilterDiffOutCoefMax=[]  ReciprocalOutMin=[]  ReciprocalOutMax=[]  SumDenOutMin=[]  SumDenOutMax=[]  SumNumOutMin=[]  SumNumOutMax=[]  DivideOutMin=[]  DivideOutMax=[]  UdiffTsProdOutMin=[]  UdiffTsProdOutMax=[]  NTsProdOutMin=[]  NTsProdOutMax=[]  UintegralTsProdOutMin=[]  UintegralTsProdOutMax=[]  UngainTsProdOutMin=[]  UngainTsProdOutMax=[]  IntegratorContinuousStateAttributes=''  IntegratorStateMustResolveToSignalObject=off  IntegratorRTWStateStorageClass=Auto  FilterContinuousStateAttributes=''  FilterStateMustResolveToSignalObject=off  FilterRTWStateStorageClass=Auto  ParallelPVariant=Disabled  IdealPVariant=Disabled  IVariant=InternalParameters  DVariant=Disabled  IntegratorVariant=Continuous  SatVariant=Disabled  AWVariant=Passthrough  PCopyVariant=Disabled  TRVariant=Disabled  FdbkBlocksVariant=Forward  IdealPFdbkVariant=Disabled  SatFdbkVariant=Disabled  DerivativeFilterVariant=Disabled  NVariant=Disabled  NCopyVariant=Disabled_SignalSpec  FilterICVariant=Disabled  IntegratorICVariant=InternalICs  ExternalResetVariant=Disabled  TRSumVariant=Passthrough  SumFdbkVariant=Disabled  SumVariant=Passthrough_I  TsampFilterVariant=InternalTs  TsampNgainVariant=Passthrough  TsampIntegralVariant=Passthrough  ExternalSaturationOutDataTypeStr=Inherit: Same as second input
  Polar to Cartesian : simulink_extras/Transformations/Polar to Cartesian
      settings: SourceProductBaseCode=SL
  Power calculation : Subsystem
  Product3 : Product
  Saturation : Saturate  UpperLimit=Imax  LowerLimit=0
  Saturation1 : Saturate  UpperLimit=0.1*Pconv  LowerLimit=-0.1*Pconv
  Saturation2 : Saturate  UpperLimit=0.1*Pconv  LowerLimit=-0.1*Pconv
  Saturation7 : Saturate  UpperLimit=0  LowerLimit=-Qmax_lvrt
  Second-Order Filter : eeGeneralControl/Second-Order Filter  FilterType=Low-pass  fn=150  Zeta=0.9  Ts=-1  A0=0  Ph0=0  f0=0  b0=0
      settings: SourceProductBaseCode=PS
  Second-Order Filter1 : eeGeneralControl/Second-Order Filter  FilterType=Low-pass  fn=10  Zeta=0.9  Ts=-1  A0=50  Ph0=0  f0=0.001  b0=50
      settings: SourceProductBaseCode=PS
  Step : Step  Commented=on  Time=0.1  After=0.3*3711  SampleTime=0
  Step1 : Step  Commented=on  Time=0.2  After=0.2*3711  SampleTime=0
  Sum{,4,6,11} (4 alike) : Sum  Inputs=|+-
  Sum2 : Sum  Inputs=-+|
  Sum3 : Sum  Inputs=|++
  Sum5 : Sum  Inputs=|++
  Switch2 : Switch  Threshold=1
  Terminator : Terminator
  iq+* : Outport
  id+* : Outport  Port=2
  iq-* : Outport  Port=3
  id-* : Outport  Port=4
  m : Outport  Port=5
  wires:
  Gain1/1 -> Integrator1/1
  Gain/1 -> Integrator/1
  NOT/1 -> Product3/2
  [iqp] -> Mux1/5
  [idp] -> Mux1/6
  [PQdq] -> Mux1/10
  [f] -> Mux1/9
  [idn] -> Mux1/8
  [iqn] -> Mux1/7
  [vdn] -> Mux1/4
  [vqn] -> Mux1/3
  [vdp] -> Mux1/2
  Constant11/1 -> Sum11/1
  Gain14/1 -> Sum11/2
  Sum11/1 -> Gain15/1
  [vqfilt] -> Gain14/1
  Saturation7/1 -> Gain16/1, Compare To Constant1/1
  Gain15/1 -> Saturation7/1
  Gain16/1 -> Switch2/1
  Compare To Constant1/1 -> [LVRT_true]
  Switch2/1 -> Cartesian to Polar/2
  Integrator1/1 -> Switch2/3
  [LVRT_true] -> Switch2/2
  [LVRT_true] -> NOT/1
  [idn] -> Power calculation/8(id-)
  [iqn] -> Power calculation/7(iq-)
  [vdn] -> Power calculation/6(vd-)
  [vqn] -> Power calculation/5(vq-)
  [vdp] -> Power calculation/2(vd+)
  [idp] -> Power calculation/4(id+)
  Power calculation/1(PQ) -> Demux/1, [PQdq]
  [iqp] -> Power calculation/3(iq+)
  [vqp] -> Power calculation/1(vq+)
  Demux2/4 -> [idn]
  Demux2/3 -> [iqn]
  Demux2/2 -> [idp]
  Demux2/1 -> [iqp]
  Demux1/4 -> [vdn]
  Demux1/3 -> [vqn]
  Demux1/2 -> [vdp]
  Demux1/1 -> [vqp], Second-Order Filter/1
  iqd+-/1 -> Demux2/1
  vqd+-/1 -> Demux1/1
  Second-Order Filter/1 -> [vqfilt]
  Sum/1 -> Gain/1
  Product3/1 -> Gain1/1
  Mux1/1 -> m/1
  [vqp] -> Mux1/1
  freq/1 -> [f]
  Blk/1 -> Terminator/1
  Integrator/1 -> Cartesian to Polar/1
  Pset/1 -> Sum3/1
  Sum2/1 -> Product3/1
  Constant2/1 -> Sum6/1
  [vqfilt] -> Sum6/2
  Gain6/1 -> Saturation2/1
  Sum6/1 -> Gain6/1
  Sum5/1 -> Sum2/2  "Qref"
  Saturation1/1 -> Sum3/2
  Sum4/1 -> Gain5/1
  Gain5/1 -> Saturation1/1
  Constant1/1 -> Sum4/1
  Sum3/1 -> Sum/1  "Pref"
  Demux/2 -> Sum2/1  "Q"
  Demux/1 -> Sum/2  "P"
  Saturation/1 -> Polar to Cartesian/1
  Cartesian to Polar/1 -> Saturation/1
  Polar to Cartesian/2 -> id+*/1
  Polar to Cartesian/1 -> iq+*/1
  Cartesian to Polar/2 -> Polar to Cartesian/2
  Qset/1 -> Sum5/1
  Saturation2/1 -> Sum5/2
  [f] -> Second-Order Filter1/1
  Second-Order Filter1/1 -> Sum4/2
  Constant9/1 -> iq-*/1
  Constant10/1 -> id-*/1

== system Scenario_3_PF/G1/VSC/VSC Control/Control loops/Phasor PQ 1st/Outer-loop ==
  note: Limits the converter current
  note: Frequency droop
  note: Voltage droop
  note: Reactive power control
  note: Active power control
  note: LVRT
  Pset : Inport
  Qset : Inport  Port=2
  vqd+- : Inport  Port=3
  iqd+- : Inport  Port=4
  freq : Inport  Port=5
  Blk : Inport  Port=6
  Cartesian to Polar : simulink_extras/Transformations/Cartesian to Polar
  Compare To Constant1 : simulink/Logic and Bit Operations/Compare To Constant  relop=<  const=0  OutDataTypeStr=boolean
  Constant1 : Constant  Value=fg
  Constant10 : Constant  Value=0
  Constant11 : Constant  Value=Vlvrt0
  Constant2 : Constant  Value=Vmvpk
  Constant9 : Constant  Value=0
  Demux1 : Demux
  Demux2 : Demux
  Divide1 : Product  Inputs=*/
  Divide2 : Product  Inputs=*/
  First-Order Filter : powerlib_meascontrol/Filters/First-Order Filter  FilterType=Lowpass  Tc=1/wpq  Ts=0  Initialize=off  Vac_Init=[0, 0, 60]  Vdc_Init=0  PlotResponse=off  FreqRange="[0,  200,  1]"
  First-Order Filter2 : powerlib_meascontrol/Filters/First-Order Filter  FilterType=Lowpass  Tc=1/wpq  Ts=0  Initialize=off  Vac_Init=[0, 0, 60]  Vdc_Init=0  PlotResponse=off  FreqRange="[0,  200,  1]"
  Gain : Gain  Gain=2/3
  Gain1 : Gain  Gain=2/3
  Gain14 : Gain  Gain=1/Vmvpk
  Gain15 : Gain  Gain=Klvrt
  Gain16 : Gain  Gain=Iconvbase
  Gain5 : Gain  Gain=-1/Kfdroop*(Pconv/fg)
  Gain6 : Gain  Gain=-1/Kvdroop*(Pconv/Vmvpk)
  Mux1 : Mux  Inputs=10
  Polar to Cartesian : simulink_extras/Transformations/Polar to Cartesian
      settings: SourceProductBaseCode=SL
  Power calculation : Subsystem
  Saturation : Saturate  UpperLimit=Imax  LowerLimit=0
  Saturation1 : Saturate  UpperLimit=0.1*Pconv  LowerLimit=-0.1*Pconv
  Saturation2 : Saturate  UpperLimit=0.1*Pconv  LowerLimit=-0.1*Pconv
  Saturation3 : Saturate  UpperLimit=inf  LowerLimit=eps
  Saturation4 : Saturate  UpperLimit=inf  LowerLimit=eps
  Saturation7 : Saturate  UpperLimit=0  LowerLimit=-Qmax_lvrt
  Second-Order Filter : eeGeneralControl/Second-Order Filter  FilterType=Low-pass  fn=150  Zeta=0.9  Ts=-1  A0=0  Ph0=0  f0=0  b0=0
      settings: SourceProductBaseCode=PS
  Second-Order Filter1 : eeGeneralControl/Second-Order Filter  FilterType=Low-pass  fn=10  Zeta=0.9  Ts=-1  A0=50  Ph0=0  f0=0.001  b0=50
      settings: SourceProductBaseCode=PS
  Step : Step  Commented=on  Time=0.1  After=0.3*3711  SampleTime=0
  Step1 : Step  Commented=on  Time=0.2  After=0.2*3711  SampleTime=0
  Sum11 : Sum  Inputs=|+-
  Sum3 : Sum  Inputs=|++
  Sum4 : Sum  Inputs=|+-
  Sum5 : Sum  Inputs=|++
  Sum6 : Sum  Inputs=|+-
  Switch2 : Switch  Threshold=1
  Terminator : Terminator
  iq+* : Outport
  id+* : Outport  Port=2
  iq-* : Outport  Port=3
  id-* : Outport  Port=4
  m : Outport  Port=5
  wires:
  [vqp] -> Saturation4/1
  Saturation4/1 -> Divide2/2
  Divide2/1 -> Gain1/1
  Gain1/1 -> First-Order Filter2/1
  Gain/1 -> First-Order Filter/1
  [vqp] -> Saturation3/1
  Divide1/1 -> Gain/1
  Saturation3/1 -> Divide1/2
  Constant10/1 -> id-*/1
  Constant9/1 -> iq-*/1
  Second-Order Filter1/1 -> Sum4/2
  [f] -> Second-Order Filter1/1
  Saturation2/1 -> Sum5/2
  Qset/1 -> Sum5/1
  Cartesian to Polar/2 -> Polar to Cartesian/2
  Polar to Cartesian/1 -> iq+*/1
  Polar to Cartesian/2 -> id+*/1
  Cartesian to Polar/1 -> Saturation/1
  Saturation/1 -> Polar to Cartesian/1
  Sum3/1 -> Divide1/1  "Pref"
  Constant1/1 -> Sum4/1
  Gain5/1 -> Saturation1/1
  Sum4/1 -> Gain5/1
  Saturation1/1 -> Sum3/2
  Sum5/1 -> Divide2/1  "Qref"
  Sum6/1 -> Gain6/1
  Gain6/1 -> Saturation2/1
  [vqfilt] -> Sum6/2
  Constant2/1 -> Sum6/1
  Pset/1 -> Sum3/1
  First-Order Filter/1 -> Cartesian to Polar/1
  Blk/1 -> Terminator/1
  freq/1 -> [f]
  [vqp] -> Mux1/1
  Mux1/1 -> m/1
  Second-Order Filter/1 -> [vqfilt]
  vqd+-/1 -> Demux1/1
  iqd+-/1 -> Demux2/1
  Demux1/1 -> Second-Order Filter/1, [vqp]
  Demux1/2 -> [vdp]
  Demux1/3 -> [vqn]
  Demux1/4 -> [vdn]
  Demux2/1 -> [iqp]
  Demux2/2 -> [idp]
  Demux2/3 -> [iqn]
  Demux2/4 -> [idn]
  [vqp] -> Power calculation/1(vq+)
  [iqp] -> Power calculation/3(iq+)
  Power calculation/1(PQ) -> [PQdq]
  [idp] -> Power calculation/4(id+)
  [vdp] -> Power calculation/2(vd+)
  [vqn] -> Power calculation/5(vq-)
  [vdn] -> Power calculation/6(vd-)
  [iqn] -> Power calculation/7(iq-)
  [idn] -> Power calculation/8(id-)
  [LVRT_true] -> Switch2/2
  First-Order Filter2/1 -> Switch2/3
  Switch2/1 -> Cartesian to Polar/2
  Compare To Constant1/1 -> [LVRT_true]
  Gain16/1 -> Switch2/1
  Gain15/1 -> Saturation7/1
  Saturation7/1 -> Compare To Constant1/1, Gain16/1
  [vqfilt] -> Gain14/1
  Sum11/1 -> Gain15/1
  Gain14/1 -> Sum11/2
  Constant11/1 -> Sum11/1
  [vdp] -> Mux1/2
  [vqn] -> Mux1/3
  [vdn] -> Mux1/4
  [iqn] -> Mux1/7
  [idn] -> Mux1/8
  [f] -> Mux1/9
  [PQdq] -> Mux1/10
  [idp] -> Mux1/6
  [iqp] -> Mux1/5

== system Scenario_3_PF/G1/VSC/VSC Control/Control loops/SW, EMT AVG, Phasor Quasi-EMT/Inner-loop ==
  note: Positive-sequence current control
  note: Negative-sequence current control
  iq+* : Inport
  id+* : Inport  Port=2
  iq-* : Inport  Port=3
  id-* : Inport  Port=4
  Blk : Inport  Port=5
  vqd+- : Inport  Port=6
  iqd+- : Inport  Port=7
  Demux1 : Demux
  Demux2 : Demux
  Gain{,1..3} (4 alike) : Gain  Gain=Xt
  NOT{,1..3} (4 alike) : Logic  Operator=NOT  IconShape=distinctive  AllPortsSameDT=off  OutDataTypeStr=boolean
  PID Controller{1..4} (4 alike) : pid_lib/PID Controller  Controller=PI  Form=Ideal  TimeDomain=Continuous-time  UseExternalTs=off  SampleTime=-1  IntegratorMethod=Forward Euler  FilterMethod=Forward Euler  ControllerParametersSource=internal  P=kp_c  I=1/ti_c  D=0  UseFilter=on  N=100  TunerSelectOption=Transfer Function Based (PID Tuner App)  InitialConditionSource=internal  InitialConditionForIntegrator=0  InitialConditionForFilter=0  DifferentiatorICPrevScaledInput=0  ExternalReset=level  TrackingMode=off  Kt=1  LimitOutput=off  SatLimitsSource=internal  UpperSaturationLimit=10*Vmvpk  LowerSaturationLimit=-10*Vmvpk  LinearizeAsGain=off  AntiWindupMode=none  Kb=1  POutMin=[]  POutMax=[]  IOutMin=[]  IOutMax=[]  DOutMin=[]  DOutMax=[]  NOutMin=[]  NOutMax=[]  SumOutMin=[]  SumOutMax=[]  SaturationOutMin=[]  SaturationOutMax=[]  PParamMin=[]  PParamMax=[]  IParamMin=[]  IParamMax=[]  DParamMin=[]  DParamMax=[]  NParamMin=[]  NParamMax=[]  KbParamMin=[]  KbParamMax=[]  KtParamMin=[]  KtParamMax=[]  KbOutMin=[]  KbOutMax=[]  KtOutMin=[]  KtOutMax=[]  IntegratorOutMin=[]  IntegratorOutMax=[]  FilterOutMin=[]  FilterOutMax=[]  SumI1OutMin=[]  SumI1OutMax=[]  SumI2OutMin=[]  SumI2OutMax=[]  SumI3OutMin=[]  SumI3OutMax=[]  SumI4OutMin=[]  SumI4OutMax=[]  SumDOutMin=[]  SumDOutMax=[]  DifferentiatorOutMin=[]  DifferentiatorOutMax=[]  FilterDiffOutCoefMin=[]  FilterDiffOutCoefMax=[]  ReciprocalOutMin=[]  ReciprocalOutMax=[]  SumDenOutMin=[]  SumDenOutMax=[]  SumNumOutMin=[]  SumNumOutMax=[]  DivideOutMin=[]  DivideOutMax=[]  UdiffTsProdOutMin=[]  UdiffTsProdOutMax=[]  NTsProdOutMin=[]  NTsProdOutMax=[]  UintegralTsProdOutMin=[]  UintegralTsProdOutMax=[]  UngainTsProdOutMin=[]  UngainTsProdOutMax=[]  IntegratorContinuousStateAttributes=''  IntegratorStateMustResolveToSignalObject=off  IntegratorRTWStateStorageClass=Auto  FilterContinuousStateAttributes=''  FilterStateMustResolveToSignalObject=off  FilterRTWStateStorageClass=Auto  ParallelPVariant=Passthrough  IdealPVariant=InternalParameters  IVariant=InternalParameters  DVariant=Disabled  IntegratorVariant=Continuous  SatVariant=Disabled  AWVariant=Passthrough  PCopyVariant=Disabled  TRVariant=Disabled  FdbkBlocksVariant=Forward  IdealPFdbkVariant=Disabled  SatFdbkVariant=Disabled  DerivativeFilterVariant=Disabled  NVariant=Disabled  NCopyVariant=Disabled_SignalSpec  FilterICVariant=Disabled  IntegratorICVariant=InternalICs  ExternalResetVariant=ExternalReset  TRSumVariant=Passthrough  SumFdbkVariant=Disabled  SumVariant=Sum_PI  TsampFilterVariant=InternalTs  TsampNgainVariant=Passthrough  TsampIntegralVariant=Passthrough  ExternalSaturationOutDataTypeStr=Inherit: Same as second input
  Product{,1..3} (4 alike) : Product
  Sum : Sum  Inputs=|+-
  Sum1 : Sum  Inputs=+-+
  Sum2 : Sum  Inputs=+--
  Sum3 : Sum  Inputs=-+|
  Sum4 : Sum  Inputs=|+-
  Sum5 : Sum  Inputs=--+
  Sum6 : Sum  Inputs=+-+
  Sum7 : Sum  Inputs=-+|
  vq+* : Outport
  vd+* : Outport  Port=2
  vq-* : Outport  Port=3
  vd-* : Outport  Port=4
  wires:
  [vdp] -> Sum1/3
  iq+*/1 -> Sum/1
  [iqp] -> Gain1/1, Sum/2
  [idp] -> Gain/1, Sum3/1
  PID Controller3/1 -> Sum1/2
  Gain1/1 -> Sum1/1
  PID Controller2/1 -> Sum2/2
  Gain/1 -> Sum2/3
  id+*/1 -> Sum3/2
  Blk/1 -> [blk]
  [blk] -> NOT/1, PID Controller2/2
  Product/1 -> PID Controller2/1
  Sum/1 -> Product/1
  NOT/1 -> Product/2
  [blk] -> PID Controller3/2, NOT1/1
  NOT1/1 -> Product1/2
  Sum3/1 -> Product1/1
  Product1/1 -> PID Controller3/1
  Sum1/1 -> vd+*/1
  Sum2/1 -> vq+*/1
  [vqp] -> Sum2/1
  Demux2/2 -> [idp]
  iqd+-/1 -> Demux2/1
  Demux2/4 -> [idn]
  Demux1/3 -> [vqn]
  Demux1/2 -> [vdp]
  Demux1/4 -> [vdn]
  Demux1/1 -> [vqp]
  Demux2/3 -> [iqn]
  Demux2/1 -> [iqp]
  vqd+-/1 -> Demux1/1
  iq-*/1 -> Sum4/1
  [blk] -> PID Controller4/2, NOT3/1
  Sum5/1 -> vd-*/1
  NOT2/1 -> Product2/2
  Sum7/1 -> Product3/1
  id-*/1 -> Sum7/2
  PID Controller4/1 -> Sum5/2
  NOT3/1 -> Product3/2
  Product3/1 -> PID Controller4/1
  PID Controller1/1 -> Sum6/2
  Product2/1 -> PID Controller1/1
  Sum4/1 -> Product2/1
  Gain3/1 -> Sum5/1
  Sum6/1 -> vq-*/1
  [blk] -> NOT2/1, PID Controller1/2
  Gain2/1 -> Sum6/3
  [idn] -> Gain2/1, Sum7/1
  [iqn] -> Sum4/2, Gain3/1
  [vqn] -> Sum6/1
  [vdn] -> Sum5/3
